simulink model "opamp_model_2014a"  (R2014a)
settings: Solver=ode45  StartTime=0.0  StopTime=10.0  RelTol=1e-3
libraries: fl_lib x10, elec_lib x3, nesl_utility x3
settings Model: CovModelRefEnable=off  CovSFcnEnable=on  Creator=Aron  LastModifiedBy=Aron
settings DataIOCC: SaveFormat=StructureWithTime
settings DebuggingCC: MergeDetectMultiDrivingBlocksExec=error  SolverPrmCheckMsg=none  FrameProcessingCompatibilityMsg=error
settings HardwareCC: ProdBitPerPointer=64  ProdLargestAtomicFloat=Float  ProdIntDivRoundTo=Zero  ProdEndianess=LittleEndian  ProdHWDeviceType=Specified
settings GRTTargetCC: GeneratePreprocessorConditionals=Use local settings

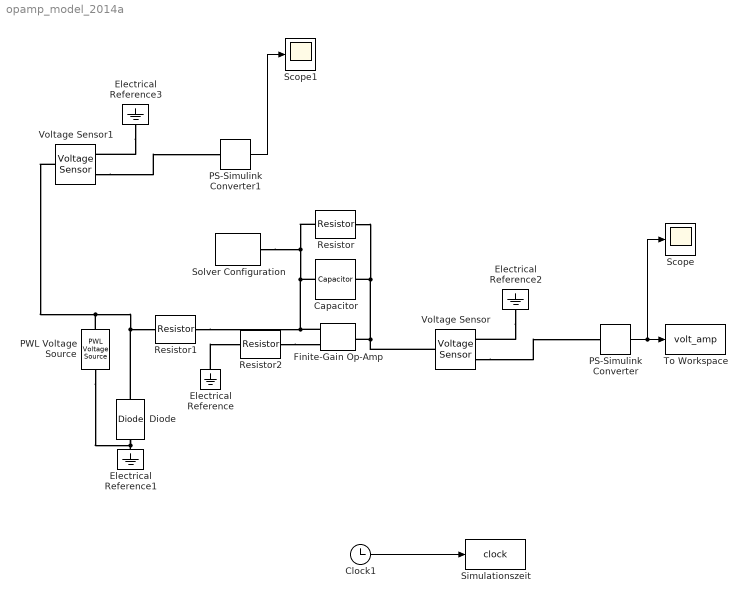
== system opamp_model_2014a ==
  Capacitor : fl_lib/Electrical/Electrical Elements/Capacitor  c=1e-10 F  r=1e-8 Ohm  g=0 1/Ohm  i_specify=off  i_priority=None  i=0 A  v_specify=off  v_priority=None  v=0 V  vc_specify=off  vc_priority=None  vc=0 V
  Clock1 : Clock
  Diode : elec_lib/Semiconductor Devices/Diode  ModelType=2  Vf=0.6 V  Ron=0.3 Ohm  Goff=1e-8 S  Rz=0.3 Ohm  Vz=50 V  C_PWL=5 pF  prmExp=1  I12=[ 0.0137 0.545 ] A  V12=[ 0.6 0.7 ] V  I1=0.0137 A  V1=0.6 V  RS=0.01 Ohm  IS=1e-12 A  Tmeas=25 C  ec=1  BV=Inf V  C_param=1  CJ0=5 pF  VJ=1 V  Mgrad=0.5  Vvec=[ 0.1 10 100 ] V  Cvec=[ 3.5 1 0.4 ] pF  FC=0.5  Q_param=1  Irrm=-7.15 A  iF=4 A  didt=-750 A/us  trr=115 ns  TT=50 ns  tau=100 ns  T_param=1  IS_T2=1.25e-7 A  I1_T2=0.245 A  V1_T2=0.5 V  Tmeas2=125 C  EG_param=1  EG=1.11 eV  XTI_param=1  XTI=3  dBVdT=0 V/K  Tdevice=25 C  Rth=[ 0 10 ] K/W  thermal_mass_parameterization=1  thermal_mass=[ 0 1 ] J/K  thermal_time_constant=[ 0 10 ] s  thermal_mass_initial_temperatures=[ 25 25 ] C
  Electrical Reference{,1..3} (4 alike) : fl_lib/Electrical/Electrical Elements/Electrical Reference
  Finite-Gain Op-Amp : elec_lib/Integrated Circuits/Finite-Gain Op-Amp  A=100000  Rin=1e6 Ohm  Rout=100 Ohm  Vmin=- 15 V  Vmax=15 V
  PS-Simulink Converter : nesl_utility/PS-Simulink Converter  PhysicalDomain=network_engine_domain  SubClassName=ps_output  LeftPortType=input  RightPortType=output  PseudoPeriodic=off  Frequencies=[]  Unit=1  AffineConversion=off
  PS-Simulink Converter1 : nesl_utility/PS-Simulink Converter  PhysicalDomain=network_engine_domain  SubClassName=ps_output  LeftPortType=input  RightPortType=output  PseudoPeriodic=off  Frequencies=[]  Unit=1  AffineConversion=off
  PWL Voltage Source : elec_lib/Additional Components/SPICE-Compatible Components/Sources/PWL Voltage Source  TIMElist=t s  VOLTlist=volt V  INTERP=3  EXTRAP=1
  Resistor : fl_lib/Electrical/Electrical Elements/Resistor  R=1000 Ohm  i_specify=off  i_priority=None  i=0 A  v_specify=off  v_priority=None  v=0 V
  Resistor1 : fl_lib/Electrical/Electrical Elements/Resistor  R=1 Ohm  i_specify=off  i_priority=None  i=0 A  v_specify=off  v_priority=None  v=0 V
  Resistor2 : fl_lib/Electrical/Electrical Elements/Resistor  R=1/1000 Ohm  i_specify=off  i_priority=None  i=0 A  v_specify=off  v_priority=None  v=0 V
  Scope : Scope
      settings: TimeRange=auto  MaxDataPoints=5000  SaveToWorkspace=off  SaveName=ScopeData  YMin=-2.79788  YMax=6.77335  SampleTime=-1
  Scope1 : Scope
      settings: TimeRange=auto  MaxDataPoints=5000  SaveToWorkspace=off  YMin=-0.0067  YMax=0.00278  SampleTime=-1
  Simulationszeit : ToWorkspace  VariableName=clock  SampleTime=-1
  Solver Configuration : nesl_utility/Solver Configuration  PhysicalDomain=network_engine_domain  SubClassName=solver  LeftPortType=input  RightPortType=generic  Accelerate=off  Tones=[]  Harmonics=[]  SimulateNoise=off  Profile=off  UseLocalSampling=off  EnableSwitchedLinearOptims=on  FrequencyDomain=off  UseCCode=off  RelTol=0.001  AbsTol=1e-06  MinStep=1e-09  ToWorkspace=off  RevertToSquareIcSolve=off  NumHomotopyIterations=100  PhasorMode=off  PhasorModeNumHarmonics=1  DoDC=off  ResidualTolerance=1e-09  UseLocalSolver=off  LocalSolverChoice=NE_BACKWARD_EULER_ADVANCER  LocalSolverSampleTime=0.001  DoFixedCost=off  MaxNonlinIter=3  MaxModeIter=2  LinearAlgebra=Full  DelaysMemoryBudget=1024  AutomaticFiltering=on  FilteringTimeConstant=0.001
  To Workspace : ToWorkspace  VariableName=volt_amp  SaveFormat=Timeseries  SampleTime=-1
  Voltage Sensor : fl_lib/Electrical/Electrical Sensors/Voltage Sensor
  Voltage Sensor1 : fl_lib/Electrical/Electrical Sensors/Voltage Sensor
  wires:
  PS-Simulink Converter/1 -> Scope/1, To Workspace/1
  Clock1/1 -> Simulationszeit/1
  PS-Simulink Converter1/1 -> Scope1/1
  connections:
  Voltage Sensor1/LConn1 -- PWL Voltage Source/LConn1 -- Diode/RConn1 -- Resistor1/LConn1
  Resistor/RConn1 -- Finite-Gain Op-Amp/RConn1 -- Voltage Sensor/LConn1 -- Capacitor/RConn1
  Electrical Reference/LConn1 -- Resistor2/LConn1
  Voltage Sensor/RConn1 -- PS-Simulink Converter/LConn1
  Electrical Reference2/LConn1 -- Voltage Sensor/RConn2
  Capacitor/LConn1 -- Resistor1/RConn1 -- Finite-Gain Op-Amp/LConn1 -- Solver Configuration/RConn1 -- Resistor/LConn1
  Resistor2/RConn1 -- Finite-Gain Op-Amp/LConn2
  Electrical Reference3/LConn1 -- Voltage Sensor1/RConn2
  Voltage Sensor1/RConn1 -- PS-Simulink Converter1/LConn1
  Electrical Reference1/LConn1 -- PWL Voltage Source/RConn1 -- Diode/LConn1
